simulink model "sharp"  (R2017a)
settings: Solver=FixedStepAuto  StartTime=0.0  StopTime=inf  RelTol=1e-3  EnableMultiTasking=on
libraries: arduinolib x5
settings Model: SimulationMode=external  ExtModeTrigDuration=2  Creator=sugato  LastModifiedBy=sugato
settings OptimizationCC: PassReuseOutputArgsThreshold=0  MaxStackSize=64
settings DebuggingCC: ParameterTunabilityLossMsg=error
settings HardwareCC: ProdBitPerInt=16  ProdBitPerPointer=16  ProdBitPerSizeT=16  ProdBitPerPtrDiffT=16  ProdLargestAtomicFloat=None  ProdWordSize=8  ProdHWDeviceType=Atmel->AVR  UseEmbeddedCoderFeatures=off  UseSimulinkCoderFeatures=off
settings SFSimCC: MATLABDynamicMemAlloc=off
settings RTWCC: SystemTargetFile=ert.tlc  HardwareBoard=Arduino Mega 2560  TLCOptions=-aInlineSetEventsForThisBaseRateFcn=TLC_FALSE -aSuppressMultiTaskScheduler=TLC_FALSE -aRateBasedStepFcn=1  TemplateMakefile=ert_default_tmf  Description=Embedded Coder  GenerateReport=on  Toolchain=Arduino AVR  BuildConfiguration=Faster Runs  LaunchReport=on
settings CodeAppCC: ForceParamTrailComments=on  OperatorAnnotations=on  MATLABSourceComments=on
settings ERTTargetCC: ERTCustomFileBanners=off  SupportContinuousTime=on  SupportNonInlinedSFcns=on  RemoveResetFunc=off  SupportVariableSizeSignals=on  ModelStepFunctionPrototypeControlCompliant=off

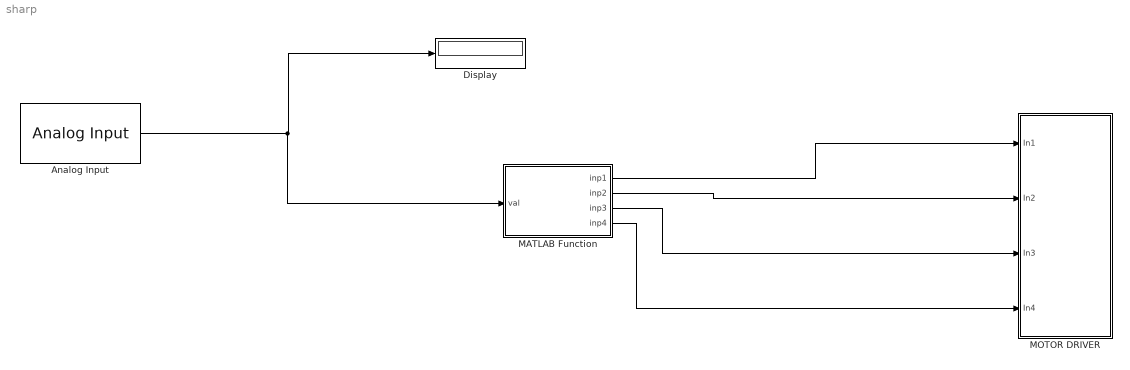
== system sharp ==
  Analog Input : arduinolib/Analog Input  pinNumber=4  sampleTime=1  blockPlatform=arduino
  Display : Display
  MATLAB Function : MATLAB Function  TreatAsAtomicUnit=on
  MOTOR DRIVER : Subsystem
  wires:
  Analog Input/1 -> MATLAB Function/1(val), Display/1
  MATLAB Function/4(inp4) -> MOTOR DRIVER/4(In4)
  MATLAB Function/1(inp1) -> MOTOR DRIVER/1(In1)
  MATLAB Function/2(inp2) -> MOTOR DRIVER/2(In2)
  MATLAB Function/3(inp3) -> MOTOR DRIVER/3(In3)

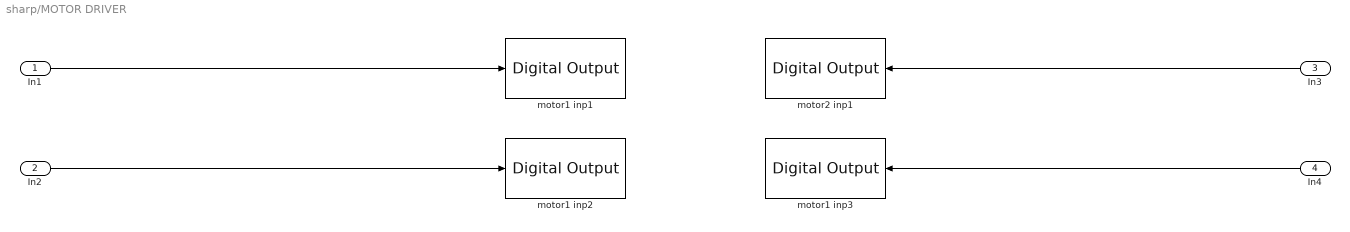
== system sharp/MOTOR DRIVER ==
  In1 : Inport
  In2 : Inport  Port=2
  In3 : Inport  Port=3
  In4 : Inport  Port=4
  motor1 inp1 : arduinolib/Digital Output  pinNumber=4  blockPlatform=arduino
  motor1 inp2 : arduinolib/Digital Output  pinNumber=6  blockPlatform=arduino
  motor1 inp3 : arduinolib/Digital Output  pinNumber=7  blockPlatform=arduino
  motor2 inp1 : arduinolib/Digital Output  pinNumber=5  blockPlatform=arduino
  wires:
  In2/1 -> motor1 inp2/1
  In1/1 -> motor1 inp1/1
  In4/1 -> motor1 inp3/1
  In3/1 -> motor2 inp1/1

== matlab function sharp/MATLAB Function ==
  data: inp1 output; inp2 output; val input; inp3 output; inp4 output
function [inp1,inp2,inp3,inp4] = input(val)
if val>=450
    % MOTOR 1
    inp1=5; % pin 4
    inp2=0; % pin 6
    
    % MOTOR 2
    inp3=0; % PIN 5
    inp4=5; % PIN 7 
    
else
     % MOTOR 1
    inp1=5;  % PIN 4
    inp2=0;  % PIN 6
    
    % MOTOR 2
    inp3=5;  % PIN 5
    inp4=0;  % PIN 7 
end

pause(0.2);
end
